simulink model "Model"  (R2023a)
settings: Solver=ode3  StartTime=0.0  StopTime=2.0  FixedStep=0.0001  RelTol=1e-3
values from neighbouring files (symbols this model uses):
  J2 = 1.26e-3    (= 0.00126)    [system_init.m]
libraries: neural x24
(part 2 of 2)

== matlab function Model/MATLAB Function ==
  settings: updateMethod=DISCRETE
  data: error input; error_output output
function error_output = fcn(error)

persistent error_filter

if isempty(error_filter)
    error_filter = 0;
end

if (error > 0)
    if (error >= 0.01)
        error_filter = error;
    else
        error_filter = 0;
    end
end

if (error < 0)
    if (abs(error) >= 0.01)
        error_filter = error;
    else
        error_filter = 0;
    end
end

if (error == 0)
    error_filter = 0;
end

error_output = error_filter;

== matlab function Model/MATLAB Function5 ==
  settings: updateMethod=DISCRETE
  data: TL input; Wmin output; beta input; dWmin_db output
function [Wmin,dWmin_db] = fcn(TL,beta)

persistent centers spreads weights bias T Time Wmin_predict dWdb

u = [TL;beta];

if isempty(centers)
    % 从数据文件加载网络参数
    data = load('RBFNN_Parameters_Wmin.mat');
    centers = data.RBF_Centers;                           % 高斯核函数中心值,2x21
    spreads = 0.84255461;                                 % 高斯核函数宽度值,标量
    weights = data.RBF_Weights;                           % 隐藏层至输出层权值,1x21
    bias = data.RBF_Bias;                                 % 输出层偏置,标量

    % 系统运行周期
    T = 0.0001;
    Time = 0;

    Wmin_predict = 0;
    dWdb = 0;
end

% 计算神经元个数
num_neurons = size(centers, 1);

% 初始化隐藏层输出数组
phi = zeros(num_neurons, 1);

% 初始化偏导数计算项数组
delta = zeros(num_neurons, 1);

if (Time > 0.8)
    % 计算隐藏层输出
    for j = 1:num_neurons
            diff = u - centers(j, :)';  % 计算输入与中心的差
            dist_sq = sum(diff .^ 2);   % 计算距离平方
            phi(j) = exp(-dist_sq / (2 * spreads^2));
            delta(j) = beta - centers(j, 2);
    end
    
    Wmin_predict = weights * phi + bias;
    dWdb = -(1 / spreads^2) * sum(weights * phi * delta);

end

Time = Time + T;

% 输出转速下降最小预测值
Wmin = Wmin_predict;

% 输出转速下降最小值关于补偿系数beta的偏导数
dWmin_db = dWdb;

end

== matlab function Model/Subsystem2/MATLAB Function7 ==
  data: TL input; y output; beta input
function y = fcn(TL,beta)

u = [TL;beta];

y = u;

== matlab function Model/RBFN_OnLineRun ==
  settings: updateMethod=DISCRETE  sampleTime=0.0001
  data: y_pred output; uk input; E output; uk_1 input; yk_1 input; yk_2 input; yk_3 input; yk_4 input; yk input; dy_duk output
function [y_pred, E, dy_duk]  = RBFN_OnLine(uk, uk_1, yk_1, yk_2, yk_3, yk_4, yk)

% 6个输入，包含当前、过去输入与过去输出
u = [uk; uk_1; yk_1; yk_2; yk_3; yk_4]; % [6 x 1]

%RBFN参数定义与初始化
persistent centers sigma W learning

if isempty(centers)
    % 从文件中加载预训练的参数，注意文件名,最好用的一组参数存在2结尾的文件里面
    data = load('RBFN_parameters2.mat');
    centers = data.centers;
    sigma = data.sigma;
    W = data.W_init;
    learning = true;
end

K = 36; % 神经元数量
H = zeros(K, 1);

% 计算偏导数
delta = zeros(K, 1); 

for j = 1:K
    % 计算第 j 个 RBF 神经元的输出
    distance = norm(u - centers(j, :)'); 
    H(j) = exp(- (distance^2) / (2 * sigma^2));

    % c_{j1} 是 centers 矩阵的第 j 行，第1个元素，也就是uk所具体对应的中心值，因为有36个神经元，所以对应36个值
    delta(j) = uk - centers(j, 1);
end

% 网络输出
y_pred = W' * H;

% 预测误差
e = yk - y_pred;
E = e;

% 学习率设置
eta_W = 0.10;    
eta_c = 0.008;    
eta_sigma = 0.005; 

epsilon = 0.001; % 误差阈值

% 判断是否需要更新参数，误差没有达到要求就更新
if learning
    W = W + eta_W * e * H;

    for j = 1:K
        centers(j, :) = centers(j, :) + ...
            eta_c * e * W(j) * H(j) * (u' - centers(j, :)) / sigma^2;
    end

    delta_sigma = 0;

    for j = 1:K
        delta_sigma = delta_sigma + ...
            e * W(j) * H(j) * (norm(u - centers(j, :)')^2) / sigma^3;
    end
    
    sigma = sigma + eta_sigma * delta_sigma / K;
end

% 收敛条件判断
if abs(e) < epsilon
    % 误差小于阈值，停止参数更新
    learning = false;
else
    % 误差大于阈值，继续参数更新
    learning = true;
end

% 计算网络输出 y 关于当前输入 u_k 的偏导数

% 推导公式：
% dy/du_k = -(1 / sigma^2) * sum_{j=1}^K [ W_j * H_j * (u_k - c_{j1})]

% 计算偏导数，计算结果是当前时刻
dy_duk = - (1 / sigma^2) * sum(W .* H .* delta);
% W_out = W;
% sigma_out = sigma;

end

== matlab function Model/calculate_for_alpha ==
  settings: updateMethod=DISCRETE
  data: error input; ya1 output; ya2 output; Ts input; ya3 output; g input; ya4 output; ya5 output; ya6 output
function [ya1, ya2, ya3, ya4, ya5, ya6]  = fcn(error, Ts, g)

persistent T time err_last err_squa err_sum err_squa_t ISE_output Err_output ISE_New ISE_Old Err_New Err_Old Ts_sum Ts_output Ts_New Ts_Old g_sum g_New g_Old g_output ITSE_New ITSE_Old ITSE_output Errt_New Errt_Old Errt_sum Errt_output
if isempty(T)
    T = 0.0001;                                        % 系统运行周期，s
    time = 0;                                          % 系统运行计时

    err_last = 0;                                      % 上一时刻误差
    err_squa = 0;                                      % 误差平方
    err_squa_t = 0;                                    % 误差平方时间加权
    err_sum = 0;                                       % 误差求和

    ISE_output = 0;                                    % ISE计算输出
    ITSE_output = 0;                                   % ITSE输出
    Err_output = 0;                                    % 误差求和输出

    ISE_New = 0;                                       % ISE新值
    ISE_Old = 0;                                       % ISE旧值

    Err_New = 0;                                       % 误差和新值
    Err_Old = 0;                                       % 误差和旧值

    Ts_sum = 0;                                        % 扭矩求和
    Ts_Old = 0;                                        % 求和旧值
    Ts_New = 0;                                        % 求和新值
    Ts_output = 0;                                     % 扭矩求和输出

    g_sum = 0;                                         % 梯度求和
    g_New = 0;                                         % 求和新值
    g_Old = 0;                                         % 求和旧值
    g_output = 0;                                      % 梯度求和输出

    ITSE_New = 0;                                      % ITSE新值
    ITSE_Old = 0;                                      % ITSE旧值

    Errt_New = 0;                                      % 误差时间加权新值
    Errt_Old = 0;                                      % 误差时间加权旧值
    Errt_output = 0;                                   % 误差时间加权输出
    Errt_sum = 0;                                      % 误差时间加权

end

if (time > 0.242)  % 运行进入稳态再计算
    if (sign(error) == sign(err_last))  % 未过零，累加需要的变量

        err_squa = err_squa + (error^2);
        err_squa_t = err_squa_t + ((error^2) * time);  % 使用时间项
        err_sum = error + err_sum;
        Errt_sum = (error * time) + Errt_sum;
        Ts_sum = Ts + Ts_sum;
        
        if(abs(error) > 0.01)
            g_sum = g + g_sum;
        else
            g_sum = g_sum;
        end

    else                                % 过零，输出上半周期结果

        ISE_New = err_squa * T;
        ITSE_New = (err_squa_t * T);
        Err_New = err_sum;
        Errt_New = Errt_sum;
        Ts_New = Ts_sum;
        g_New = g_sum;

        ISE_output = ISE_New * 0.8 + ISE_Old * 0.20;
        ITSE_output = ITSE_New * 0.74 + ITSE_Old * 0.26;
        Err_output = Err_New * 0.8 + Err_Old * 0.2;
        Errt_output = Errt_New * 0.7 + Errt_Old * 0.3;
        Ts_output = Ts_New * 0.68 + Ts_Old * 0.32;
        g_output = g_New * 0.8 + g_Old * 0.2;

        err_squa = 0;
        err_squa_t = 0;
        err_sum = 0;
        Errt_sum = 0;
        Ts_sum = 0;

        if(abs(error) > 0.01)
            g_sum = 0;
        else
            g_sum = g_sum;
        end

    end
end

% 数据传递
time = time + T;
err_last = error;

ISE_Old = ISE_output;
ITSE_Old = ITSE_output;
Err_Old = Err_output;
Errt_Old = Errt_output;
Ts_Old = Ts_output;
g_Old = g_output;

% 小数位控制
ISE_output = round(ISE_output*1000)/1000;
ITSE_output = round(ITSE_output*1000)/1000;
Err_output = round(Err_output*1000)/1000;
Errt_output = round(Errt_output*1000)/1000;
Ts_output = round(Ts_output*1000)/1000;
g_output = round(g_output*1000)/1000; 

% 结果输出
ya1 = ISE_output;                                       % 半个谐振周期ISE
ya2 = Err_output;                                       % 半个谐振周期误差和
ya3 = Ts_output;                                        % 半个谐振周期扭矩和
ya4 = g_output;                                         % 半个谐振周期梯度和
ya5 = ITSE_output;                                      % 半个谐振周期ITSE
ya6 = Errt_output;                                      % 半个谐振周期时间加权误差和

== matlab function Model/MATLAB Function1 ==
  settings: updateMethod=DISCRETE  sampleTime=0.0001
  data: e input; Sumerr output; systime output
function [Sumerr, systime] = calculate_err(e)

persistent T time Err M ErrOut Err_1

if isempty(T)
    T = 0.0001;
    time = 0;
    Err = 0;
    M = 0;
    ErrOut = 0;
    Err_1 = 0;
end

if (time > 1)

    Err = Err_1 + e;
    M = M + 1;
    Err_1 = Err;

    if (M == 10)
        ErrOut = Err*0.9 + ErrOut*0.1;
        Err = 0;
        Err_1 = 0;
        M = 0;
    end

end

time = time + T;

Sumerr = round(ErrOut*1000)/1000;
systime = time;

end

== matlab function Model/MATLAB Function2 ==
  settings: updateMethod=DISCRETE  sampleTime=0.0001
  data: dydu input; Sumdydu output
function Sumdydu = calculate_dydu(dydu)

persistent T time dydu_sum M dyduOut

if isempty(T)
    T = 0.0001;
    time = 0;
    dydu_sum = 0;
    M = 0;
    dyduOut = 0;
end

if (time > 1)

    dydu_sum = dydu_sum + dydu;
    M = M + 1;

    if (M == 10)
        % 低通滤波，取70%当前值和30%的历史值
        dyduOut = dyduOut*0.3 + dydu_sum*0.7;
        dydu_sum = 0;
        M = 0;
    end

end

time = time + T;

Sumdydu = round(dyduOut*1000)/1000;

end

== matlab function Model/MATLAB Function3 ==
  settings: updateMethod=DISCRETE  sampleTime=0.0001
  data: Tsk input; SumTs output
function SumTs = calculate_Ts(Tsk)

persistent T time Ts_sum M TsOut

if isempty(T)
    T = 0.0001;
    time = 0;
    Ts_sum = 0;
    M = 0;
    TsOut = 0;
end

if (time > 1)

    Ts_sum = Ts_sum + Tsk;
    M = M + 1;

    if (M == 10)
        % 低通滤波，取70%当前值和30%的历史值
        TsOut = TsOut*0.3 + Ts_sum*0.7;
        Ts_sum = 0;
        M = 0;
    end

end

time = time + T;

SumTs = round(TsOut*1000)/1000;

end

== matlab function Model/MATLAB Function4 ==
  settings: updateMethod=DISCRETE
  data: ISE input; a output; e input; dydu input; Ts input; J2 input
function a = calculate_a(ISE,e,dydu,Ts,J2)
persistent T time a_now a_old eta_a1 eta_a2 cnt

if isempty(T)
    T = 0.0001;
    time = 0;
    a_old = 0.0;
    a_now = 0.0;
    cnt = 0;
    % eta_a1 = 0.500;   % 评价函数为ISE+ITSE的学习率，要小一点
    % eta_a1 = 0.740;     % 评价函数为ITSE的学习率，要大一点
    eta_a1 = 0.550;     % 评价函数为ISE的学习率，要大一点
    % eta_a2 = 0.500;   % 评价函数为ISE+ITSE的学习率，要小一点
    % eta_a2 = 0.740;     % 评价函数为ITSE的学习率，要大一点
    eta_a2 = 0.550;     % 评价函数为ISE的学习率，要大一点
end

if (time >= 1.200 && cnt > 5)
    if (ISE > 0.005)
        if(J2 == 1.26e-3)
            % a_now = a_old - eta_a1 * ((2 * ISE * e * dydu * Ts) + (2 * ITSE * et * dydu * Ts));     % 评价函数为ISE+ITSE
            % a_now = a_old - eta_a1 * ((2 * ITSE * et * dydu * Ts));                                   % 评价函数为ITSE
            a_now = a_old - eta_a1 * ((2 * ISE * e * dydu * Ts));
            if (a_now > 1.2)
                a_now = 1.2;
            end

            if (a_now < 0)
                a_now = abs(a_now);
                if (a_now >1.2)
                    a_now = 1.2;
                end
            end
        end
        if(J2 == 4.35e-3)
            % a_now = a_old - eta_a2 * ((2 * ISE * e * dydu * Ts) + (2 * ITSE * et * dydu * Ts));   % 评价函数为ISE+ITSE
            % a_now = a_old - eta_a2 * ((2 * ITSE * et * dydu * Ts));                                 % 评价函数为ITSE
            a_now = a_old - eta_a2 * ((2 * ISE * e * dydu * Ts));
            if (a_now > 1.2)
                a_now = 1.2;
            end

            if (a_now < 0)
                a_now = abs(a_now);
                if (a_now >1.2)
                    a_now = 1.2;
                end
            end
        end
    else
        a_now = a_old;
    end
    cnt = 0;
end

time = time + T;
cnt = cnt + 1;

% a = a_now;
% a_old = a;

if (a_now < a_old)
    a = a_old;
% elseif (a_now - a_old < 0.01)
%     a = a_old;
else
    a = a_now;
end

a_old = a;

end
